simulink model "quality_check"  (Simulink 8.0)
settings: Solver=ode45  StartTime=0.0  StopTime=10  RelTol=1e-3
libraries: simulink x1
settings Model: Creator=Tran Minh Luan  LastModifiedBy=Tran Minh Luan

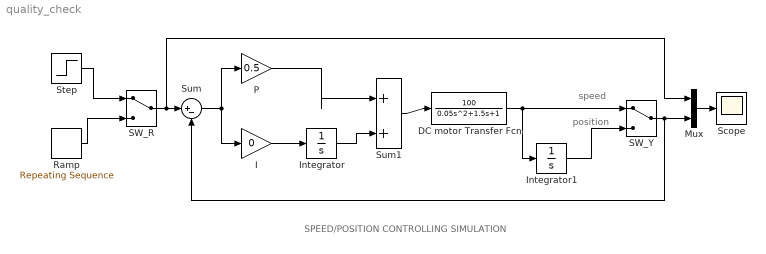
== system quality_check ==
  note: SPEED/POSITION CONTROLLING SIMULATION
  note: position
  note: speed
  DC motor Transfer Fcn : TransferFcn  Numerator=[100]  Denominator=[0.05 1.5 1]
  I : Gain  Gain=0
  Integrator : Integrator
  Integrator1 : Integrator
  Mux : Mux  Inputs=2
  P : Gain  Gain=0.5
  Ramp : simulink/Sources/Repeating Sequence  rep_seq_t=[0 10]  rep_seq_y=[0 800]
  SW_R : ManualSwitch
  SW_Y : ManualSwitch
  Scope : Scope
  Step : Step  Time=0  After=1000  SampleTime=0
  Sum : Sum  Inputs=|+-
  Sum1 : Sum  Inputs=|++
  wires:
  Step/1 -> SW_R/1
  Ramp/1 -> SW_R/2
  SW_R/1 -> Mux/1, Sum/1
  Sum/1 -> I/1, P/1
  I/1 -> Integrator/1
  P/1 -> Sum1/1
  Integrator/1 -> Sum1/2
  DC motor Transfer Fcn/1 -> Integrator1/1, SW_Y/1
  Sum1/1 -> DC motor Transfer Fcn/1
  Integrator1/1 -> SW_Y/2
  SW_Y/1 -> Sum/2, Mux/2
  Mux/1 -> Scope/1
